simulink model "sim1"  (R2019a)
settings: Solver=FixedStepAuto  StartTime=0.0  StopTime=300  FixedStep=T_s  RelTol=1e-3
undefined symbols (not defined in the file): a1, A1, a2, A2, desireValue, g, h1, h2, Km, rho
settings Model: Creator=lindt  LastModifiedBy=lindt

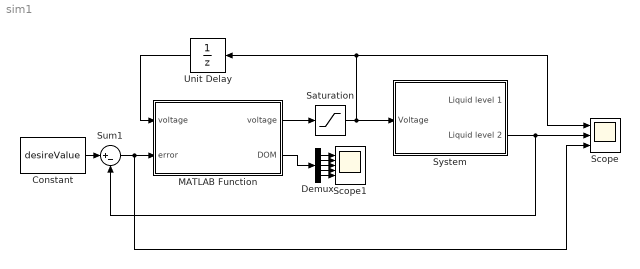
== system sim1 ==
  Constant : Constant  Value=desireValue
  Demux : Demux  Outputs=5
  MATLAB Function : MATLAB Function  TreatAsAtomicUnit=on
  Saturation : Saturate  UpperLimit=50  LowerLimit=0
  Scope : Scope  NumInputPorts=3
  Scope1 : Scope  NumInputPorts=5
  Sum1 : Sum  Inputs=|+-
  System : Subsystem
  Unit Delay : UnitDelay  SampleTime=-1  HasFrameUpgradeWarning=on
  wires:
  System/2(Liquid level 2) -> Scope/2, Sum1/2
  MATLAB Function/1(voltage) -> Saturation/1
  Demux/1 -> Scope1/1
  Demux/2 -> Scope1/2
  Demux/3 -> Scope1/3
  Demux/4 -> Scope1/4
  Demux/5 -> Scope1/5
  MATLAB Function/2(DOM) -> Demux/1
  Unit Delay/1 -> MATLAB Function/1("voltage ")
  Saturation/1 -> System/1(Voltage), Scope/1, Unit Delay/1
  Sum1/1 -> MATLAB Function/2(error), Scope/3
  Constant/1 -> Sum1/1

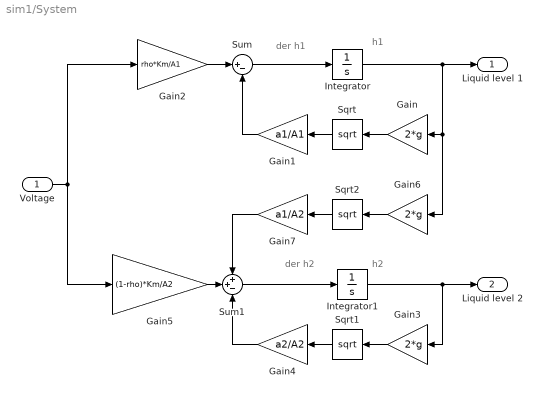
== system sim1/System ==
  note: der h1
  note: h1
  note: der h2
  note: h2
  Voltage : Inport
  Gain : Gain  Gain=2*g
  Gain1 : Gain  Gain=a1/A1
  Gain2 : Gain  Gain=rho*Km/A1
  Gain3 : Gain  Gain=2*g
  Gain4 : Gain  Gain=a2/A2
  Gain5 : Gain  Gain=(1-rho)*Km/A2
  Gain6 : Gain  Gain=2*g
  Gain7 : Gain  Gain=a1/A2
  Integrator : Integrator  InitialCondition=h1
  Integrator1 : Integrator  InitialCondition=h2
  Sqrt : Sqrt  SaturateOnIntegerOverflow=on
  Sqrt1 : Sqrt  SaturateOnIntegerOverflow=on
  Sqrt2 : Sqrt  SaturateOnIntegerOverflow=on
  Sum : Sum  Inputs=|+-
  Sum1 : Sum  Inputs=++-
  Liquid level 1 : Outport
  Liquid level 2 : Outport  Port=2
  wires:
  Gain4/1 -> Sum1/3
  Integrator1/1 -> Gain3/1, Liquid level 2/1
  Sqrt/1 -> Gain1/1
  Sqrt1/1 -> Gain4/1
  Gain6/1 -> Sqrt2/1
  Gain2/1 -> Sum/1
  Gain1/1 -> Sum/2
  Integrator/1 -> Gain6/1, Gain/1, Liquid level 1/1
  Gain7/1 -> Sum1/1
  Sqrt2/1 -> Gain7/1
  Sum/1 -> Integrator/1
  Voltage/1 -> Gain5/1, Gain2/1
  Gain3/1 -> Sqrt1/1
  Gain/1 -> Sqrt/1
  Gain5/1 -> Sum1/2
  Sum1/1 -> Integrator1/1

== matlab function sim1/MATLAB Function ==
  data: voltage input; error input; voltage output; DOM output
function [voltage, DOM]= FuzzyController(voltage, error)

DOM = [0 0 0 0 0];

inputSet = [-10 -5 0 5 10];
outSet = [-4 -2 0 2 4];

if error <= inputSet(2)
    DOM(1) = 1 - (error-inputSet(1))/(inputSet(2)-inputSet(1));
    if DOM(1) > 1
        DOM(1) = 1;
    end
    voltage = voltage + DOM(1)*outSet(1);
end

if error > inputSet(1) && error <= inputSet(3)  
    if error <= inputSet(2)
        DOM(2) = (error-inputSet(1))/(inputSet(2)-inputSet(1));
    else
        DOM(2) = 1 - (error-inputSet(2))/(inputSet(3)-inputSet(2));
    end
    voltage = voltage + DOM(2)*outSet(2);
end

if   error > inputSet(2) && error <= inputSet(4)
    if error <= inputSet(3)
        DOM(3) = (error-inputSet(2))/(inputSet(3)-inputSet(2));
    else
        DOM(3) = 1 - (error - inputSet(3))/(inputSet(4)-inputSet(3));
    end
    voltage = voltage + DOM(3)*outSet(3);
end

if error > inputSet(3) &&  error <= inputSet(5)
    if error <= inputSet(4)
        DOM(4) = (error-inputSet(3))/(inputSet(4)-inputSet(3));
    else
        DOM(4) = 1 - (error-inputSet(4))/(inputSet(5)-inputSet(4));
    end
    voltage = voltage + DOM(4)*outSet(4);
end

if error > inputSet(4)
    DOM(5) = (error-inputSet(4))/(inputSet(5)-inputSet(4));
    if DOM(5) > 1
        DOM(5) = 1;
    end
    voltage = voltage + DOM(5)*outSet(5);
end
